simulink model "robot"  (R2021b)
settings: Solver=VariableStepAuto  StartTime=0.0  StopTime=10.0  RelTol=1e-3
settings Model: Creator=nose  LastModifiedBy=nose

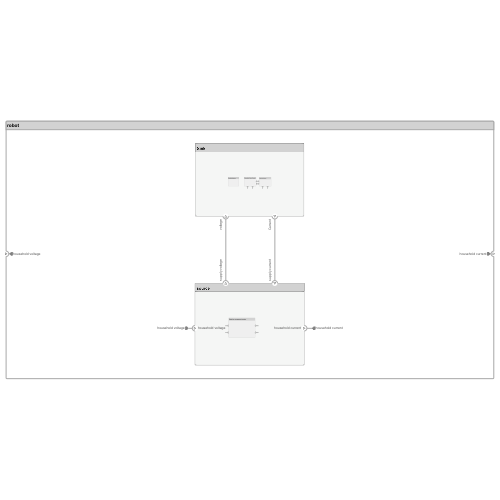
[thumbnail: Simulink's stored preview of the top-level diagram]
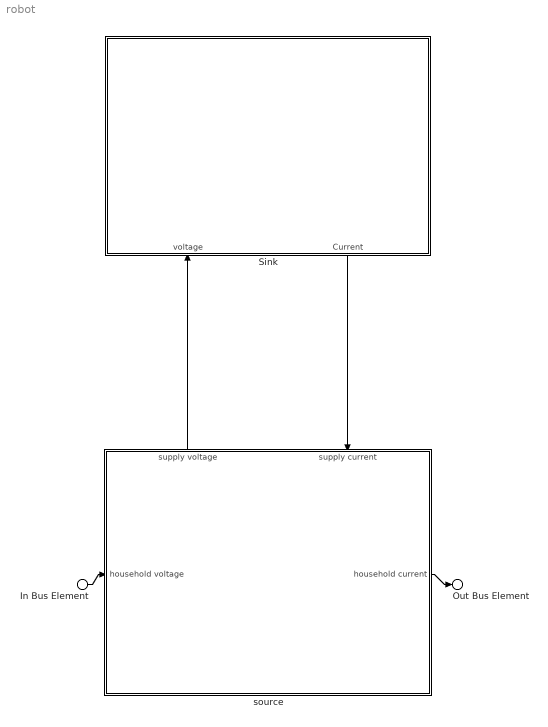
== system robot ==
  In Bus Element : Inport  PortName=household voltage
  Sink : Subsystem
      settings: PortSchema="{\"entries\":[{\"content\":{\"headerSize\":26,\"margin\":15,\"minimumSpacing\":25,\"sides\":[{\"content\":{\"connectorIds\":[]},\"type\":\"ConnectorPlacement.EquallySpacedRectSide\",\"uuid\":\"cce8d1cc-6771-426c-a0de-23a5c058ae44\"},{\"content\":{\"connectorIds\":[],\"side\":\"RIGHT\"},\"type\":\"ConnectorPlacement.EquallySpacedRectSide\",\"uuid\":\"57c46e29-2934-445f-8a04-6ff3f7f4d8fe\"},{\"content\":{\"connectorIds\":[],\"side\":\"TOP\"},\"type\":\"ConnectorPlacement.EquallySpacedRectSide\",\"uuid\":\"eb7067c1-d55e-4ae9-8630-454649e8da1e\"},{\"content\":{\"connectorIds\":[\"In1\",\"Out1\"],\"side\":\"BOTTOM\"},\"type\":\"ConnectorPlacement.EquallySpacedRectSide\",\"uuid\":\"bc61e0b0-20e7-4f9c-89f5-67eb8e0015e0\"}]},\"type\":\"ConnectorPlacement.EquallySpacedConnector\",\"uuid\":\"1a3d1b89-b469-44fc-bf92-2227b5eeb5a6\"}],\"packageUris\":[\"http://schema.mathworks.com/mf0/Connector/R2020b\"],\"version\":\"1.0\"}"
  source : Subsystem
      settings: PortSchema="{\"entries\":[{\"content\":{\"headerSize\":26,\"margin\":15,\"minimumSpacing\":25,\"sides\":[{\"content\":{\"connectorIds\":[\"In2\"]},\"type\":\"ConnectorPlacement.EquallySpacedRectSide\",\"uuid\":\"ab86f7c5-15df-4aa4-a70b-4ed2f79f5c32\"},{\"content\":{\"connectorIds\":[\"Out2\"],\"side\":\"RIGHT\"},\"type\":\"ConnectorPlacement.EquallySpacedRectSide\",\"uuid\":\"f1963fa8-65f4-4463-a82d-b8789b675b03\"},{\"content\":{\"connectorIds\":[\"Out1\",\"In1\"],\"side\":\"TOP\"},\"type\":\"ConnectorPlacement.EquallySpacedRectSide\",\"uuid\":\"01db5666-12b9-44bb-bd5a-5c24c4f58114\"}]},\"type\":\"ConnectorPlacement.EquallySpacedConnector\",\"uuid\":\"46f17ec4-de72-4b29-af46-4a561b3ef7e3\"}],\"packageUris\":[\"http://schema.mathworks.com/mf0/Connector/R2020b\"],\"version\":\"1.0\"}"
  Out Bus Element : Outport  PortName=household current
  wires:
  source/1(supply voltage) -> Sink/1(voltage)
  Sink/1(Current) -> source/1(supply current)
  In Bus Element/1 -> source/2(household voltage)
  source/2(household current) -> Out Bus Element/1

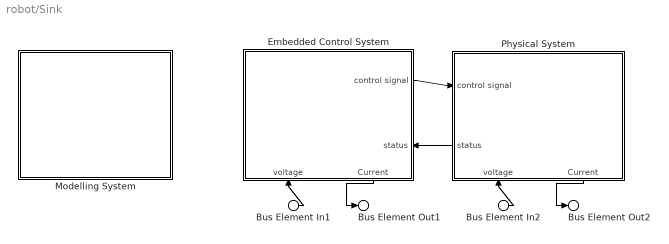
== system robot/Sink ==
  Bus Element In1 : Inport  PortName=voltage  Element=control
  Bus Element In2 : Inport  PortName=voltage  Element=physical
  Embedded Control System : Subsystem
      settings: PortSchema="{\"entries\":[{\"content\":{\"headerSize\":26,\"margin\":15,\"minimumSpacing\":25,\"sides\":[{\"content\":{\"connectorIds\":[]},\"type\":\"ConnectorPlacement.EquallySpacedRectSide\",\"uuid\":\"cce8d1cc-6771-426c-a0de-23a5c058ae44\"},{\"content\":{\"connectorIds\":[\"Out1\",\"In1\"],\"side\":\"RIGHT\"},\"type\":\"ConnectorPlacement.EquallySpacedRectSide\",\"uuid\":\"57c46e29-2934-445f-8a04-6ff3f7f4d8fe\"},{\"content\":{\"connectorIds\":[],\"side\":\"TOP\"},\"type\":\"ConnectorPlacement.EquallySpacedRectSide\",\"uuid\":\"eb7067c1-d55e-4ae9-8630-454649e8da1e\"},{\"content\":{\"connectorIds\":[\"In2\",\"Out2\"],\"side\":\"BOTTOM\"},\"type\":\"ConnectorPlacement.EquallySpacedRectSide\",\"uuid\":\"13b887ef-efdd-4ebb-88f0-3b7172777dfc\"}]},\"type\":\"ConnectorPlacement.EquallySpacedConnector\",\"uuid\":\"1a3d1b89-b469-44fc-bf92-2227b5eeb5a6\"}],\"packageUris\":[\"http://schema.mathworks.com/mf0/Connector/R2020b\"],\"version\":\"1.0\"}"
  Modelling System : Subsystem
      settings: PortSchema="{\"entries\":[{\"content\":{\"headerSize\":26,\"margin\":15,\"minimumSpacing\":25,\"sides\":[{\"content\":{\"connectorIds\":[]},\"type\":\"ConnectorPlacement.EquallySpacedRectSide\",\"uuid\":\"cce8d1cc-6771-426c-a0de-23a5c058ae44\"},{\"content\":{\"connectorIds\":[],\"side\":\"RIGHT\"},\"type\":\"ConnectorPlacement.EquallySpacedRectSide\",\"uuid\":\"57c46e29-2934-445f-8a04-6ff3f7f4d8fe\"},{\"content\":{\"connectorIds\":[],\"side\":\"TOP\"},\"type\":\"ConnectorPlacement.EquallySpacedRectSide\",\"uuid\":\"eb7067c1-d55e-4ae9-8630-454649e8da1e\"}]},\"type\":\"ConnectorPlacement.EquallySpacedConnector\",\"uuid\":\"1a3d1b89-b469-44fc-bf92-2227b5eeb5a6\"}],\"packageUris\":[\"http://schema.mathworks.com/mf0/Connector/R2020b\"],\"version\":\"1.0\"}"
  Physical System : Subsystem
      settings: PortSchema="{\"entries\":[{\"content\":{\"headerSize\":26,\"margin\":15,\"minimumSpacing\":25,\"sides\":[{\"content\":{\"connectorIds\":[\"In1\",\"Out1\"]},\"type\":\"ConnectorPlacement.EquallySpacedRectSide\",\"uuid\":\"cce8d1cc-6771-426c-a0de-23a5c058ae44\"},{\"content\":{\"connectorIds\":[],\"side\":\"RIGHT\"},\"type\":\"ConnectorPlacement.EquallySpacedRectSide\",\"uuid\":\"57c46e29-2934-445f-8a04-6ff3f7f4d8fe\"},{\"content\":{\"connectorIds\":[],\"side\":\"TOP\"},\"type\":\"ConnectorPlacement.EquallySpacedRectSide\",\"uuid\":\"eb7067c1-d55e-4ae9-8630-454649e8da1e\"},{\"content\":{\"connectorIds\":[\"In2\",\"Out2\"],\"side\":\"BOTTOM\"},\"type\":\"ConnectorPlacement.EquallySpacedRectSide\",\"uuid\":\"76e84532-edcd-4bc8-b0e9-3aa90831f893\"}]},\"type\":\"ConnectorPlacement.EquallySpacedConnector\",\"uuid\":\"1a3d1b89-b469-44fc-bf92-2227b5eeb5a6\"}],\"packageUris\":[\"http://schema.mathworks.com/mf0/Connector/R2020b\"],\"version\":\"1.0\"}"
  Bus Element Out1 : Outport  PortName=Current  Element=control
  Bus Element Out2 : Outport  PortName=Current  Element=physical
  wires:
  Bus Element In1/1 -> Embedded Control System/2(voltage)
  Bus Element In2/1 -> Physical System/2(voltage)
  Embedded Control System/2(Current) -> Bus Element Out1/1
  Physical System/2(Current) -> Bus Element Out2/1
  Embedded Control System/1(control signal) -> Physical System/1(control signal)
  Physical System/1(status) -> Embedded Control System/1(status)

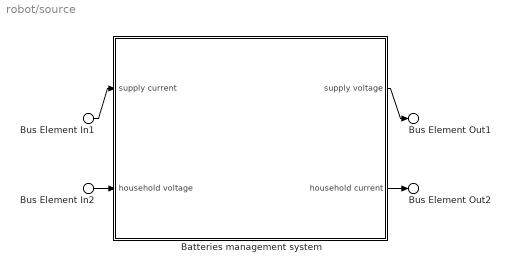
== system robot/source ==
  Bus Element In1 : Inport  PortName=supply current
  Bus Element In2 : Inport  Port=2  PortName=household voltage
  Batteries management system : Subsystem
      settings: PortSchema="{\"entries\":[{\"content\":{\"headerSize\":26,\"margin\":15,\"minimumSpacing\":25,\"sides\":[{\"content\":{\"connectorIds\":[\"In1\",\"In2\"]},\"type\":\"ConnectorPlacement.EquallySpacedRectSide\",\"uuid\":\"ab86f7c5-15df-4aa4-a70b-4ed2f79f5c32\"},{\"content\":{\"connectorIds\":[\"Out2\",\"Out1\"],\"side\":\"RIGHT\"},\"type\":\"ConnectorPlacement.EquallySpacedRectSide\",\"uuid\":\"f1963fa8-65f4-4463-a82d-b8789b675b03\"},{\"content\":{\"connectorIds\":[],\"side\":\"TOP\"},\"type\":\"ConnectorPlacement.EquallySpacedRectSide\",\"uuid\":\"01db5666-12b9-44bb-bd5a-5c24c4f58114\"},{\"content\":{\"connectorIds\":[],\"side\":\"BOTTOM\"},\"type\":\"ConnectorPlacement.EquallySpacedRectSide\",\"uuid\":\"ad04bc5b-bf31-4298-9687-69f53933a826\"}]},\"type\":\"ConnectorPlacement.EquallySpacedConnector\",\"uuid\":\"46f17ec4-de72-4b29-af46-4a561b3ef7e3\"}],\"packageUris\":[\"http://schema.mathworks.com/mf0/Connector/R2020b\"],\"version\":\"1.0\"}"
  Bus Element Out1 : Outport  PortName=supply voltage
  Bus Element Out2 : Outport  Port=2  PortName=household current
  wires:
  Bus Element In1/1 -> Batteries management system/1(supply current)
  Batteries management system/2(supply voltage) -> Bus Element Out1/1
  Bus Element In2/1 -> Batteries management system/2(household voltage)
  Batteries management system/1(household current) -> Bus Element Out2/1

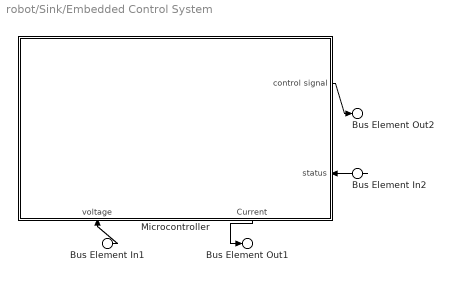
== system robot/Sink/Embedded Control System ==
  Bus Element In2 : Inport  PortName=status
  Bus Element In1 : Inport  Port=2  PortName=voltage
  Microcontroller : Subsystem
      settings: PortSchema="{\"entries\":[{\"content\":{\"headerSize\":26,\"margin\":15,\"minimumSpacing\":25,\"sides\":[{\"content\":{\"connectorIds\":[]},\"type\":\"ConnectorPlacement.EquallySpacedRectSide\",\"uuid\":\"bdb45843-8dc8-4990-9bf3-624b48549b20\"},{\"content\":{\"connectorIds\":[\"Out2\",\"In2\"],\"side\":\"RIGHT\"},\"type\":\"ConnectorPlacement.EquallySpacedRectSide\",\"uuid\":\"0a73e1fb-4df2-4d5d-a61e-038e5c52e735\"},{\"content\":{\"connectorIds\":[],\"side\":\"TOP\"},\"type\":\"ConnectorPlacement.EquallySpacedRectSide\",\"uuid\":\"48b402de-12bd-4d2a-b9ce-c931ca0ce21c\"},{\"content\":{\"connectorIds\":[\"In1\",\"Out1\"],\"side\":\"BOTTOM\"},\"type\":\"ConnectorPlacement.EquallySpacedRectSide\",\"uuid\":\"c7ff1f7c-598d-4839-a261-d2e7959d2121\"}]},\"type\":\"ConnectorPlacement.EquallySpacedConnector\",\"uuid\":\"51fa05e7-43b8-43a9-952b-69997c969bcd\"}],\"packageUris\":[\"http://schema.mathworks.com/mf0/Connector/R2020b\"],\"version\":\"1.0\"}"
  Bus Element Out2 : Outport  PortName=control signal
  Bus Element Out1 : Outport  Port=2  PortName=Current
  wires:
  Bus Element In2/1 -> Microcontroller/2(status)
  Microcontroller/2(control signal) -> Bus Element Out2/1
  Bus Element In1/1 -> Microcontroller/1(voltage)
  Microcontroller/1(Current) -> Bus Element Out1/1

== system robot/Sink/Modelling System ==

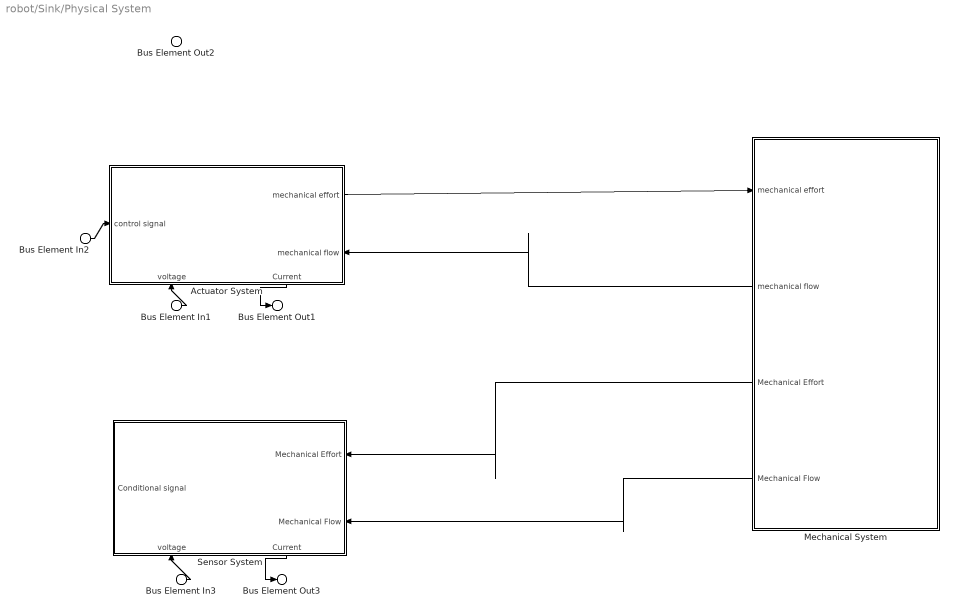
== system robot/Sink/Physical System ==
  Bus Element In2 : Inport  PortName=control signal
  Bus Element In1 : Inport  Port=2  PortName=voltage  Element=actuator
  Bus Element In3 : Inport  Port=2  PortName=voltage  Element=sensor
  Actuator System : Subsystem
      settings: PortSchema="{\"entries\":[{\"content\":{\"headerSize\":26,\"margin\":15,\"minimumSpacing\":25,\"sides\":[{\"content\":{\"connectorIds\":[\"In2\"]},\"type\":\"ConnectorPlacement.EquallySpacedRectSide\",\"uuid\":\"cce8d1cc-6771-426c-a0de-23a5c058ae44\"},{\"content\":{\"connectorIds\":[\"Out2\",\"In3\"],\"side\":\"RIGHT\"},\"type\":\"ConnectorPlacement.EquallySpacedRectSide\",\"uuid\":\"57c46e29-2934-445f-8a04-6ff3f7f4d8fe\"},{\"content\":{\"connectorIds\":[],\"side\":\"TOP\"},\"type\":\"ConnectorPlacement.EquallySpacedRectSide\",\"uuid\":\"eb7067c1-d55e-4ae9-8630-454649e8da1e\"},{\"content\":{\"connectorIds\":[\"In1\",\"Out1\"],\"side\":\"BOTTOM\"},\"type\":\"ConnectorPlacement.EquallySpacedRectSide\",\"uuid\":\"e184a07b-f7e7-418f-a075-a6148e69a320\"}]},\"type\":\"ConnectorPlacement.EquallySpacedConnector\",\"uuid\":\"1a3d1b89-b469-44fc-bf92-2227b5eeb5a6\"}],\"packageUris\":[\"http://schema.mathworks.com/mf0/Connector/R2020b\"],\"version\":\"1.0\"}"
  Mechanical System : Subsystem
      settings: PortSchema="{\"entries\":[{\"content\":{\"headerSize\":26,\"margin\":15,\"minimumSpacing\":25,\"sides\":[{\"content\":{\"connectorIds\":[\"In1\",\"Out1\",\"Out2\",\"Out3\"]},\"type\":\"ConnectorPlacement.EquallySpacedRectSide\",\"uuid\":\"cce8d1cc-6771-426c-a0de-23a5c058ae44\"},{\"content\":{\"connectorIds\":[],\"side\":\"RIGHT\"},\"type\":\"ConnectorPlacement.EquallySpacedRectSide\",\"uuid\":\"57c46e29-2934-445f-8a04-6ff3f7f4d8fe\"},{\"content\":{\"connectorIds\":[],\"side\":\"TOP\"},\"type\":\"ConnectorPlacement.EquallySpacedRectSide\",\"uuid\":\"eb7067c1-d55e-4ae9-8630-454649e8da1e\"},{\"content\":{\"connectorIds\":[],\"side\":\"BOTTOM\"},\"type\":\"ConnectorPlacement.EquallySpacedRectSide\",\"uuid\":\"4708bf5e-c359-4b7b-a4d3-6301d6aaf289\"}]},\"type\":\"ConnectorPlacement.EquallySpacedConnector\",\"uuid\":\"1a3d1b89-b469-44fc-bf92-2227b5eeb5a6\"}],\"packageUris\":[\"http://schema.mathworks.com/mf0/Connector/R2020b\"],\"version\":\"1.0\"}"
  Sensor System : Subsystem
      settings: PortSchema="{\"entries\":[{\"content\":{\"headerSize\":26,\"margin\":15,\"minimumSpacing\":25,\"sides\":[{\"content\":{\"connectorIds\":[\"Out1\"]},\"type\":\"ConnectorPlacement.EquallySpacedRectSide\",\"uuid\":\"cce8d1cc-6771-426c-a0de-23a5c058ae44\"},{\"content\":{\"connectorIds\":[\"In1\",\"In2\"],\"side\":\"RIGHT\"},\"type\":\"ConnectorPlacement.EquallySpacedRectSide\",\"uuid\":\"57c46e29-2934-445f-8a04-6ff3f7f4d8fe\"},{\"content\":{\"connectorIds\":[],\"side\":\"TOP\"},\"type\":\"ConnectorPlacement.EquallySpacedRectSide\",\"uuid\":\"eb7067c1-d55e-4ae9-8630-454649e8da1e\"},{\"content\":{\"connectorIds\":[\"In3\",\"Out2\"],\"side\":\"BOTTOM\"},\"type\":\"ConnectorPlacement.EquallySpacedRectSide\",\"uuid\":\"956056ff-9723-44b8-9837-a0ccb26e421f\"}]},\"type\":\"ConnectorPlacement.EquallySpacedConnector\",\"uuid\":\"1a3d1b89-b469-44fc-bf92-2227b5eeb5a6\"}],\"packageUris\":[\"http://schema.mathworks.com/mf0/Connector/R2020b\"],\"version\":\"1.0\"}"
  Bus Element Out2 : Outport  PortName=status
  Bus Element Out1 : Outport  Port=2  PortName=Current  Element=actuator
  Bus Element Out3 : Outport  Port=2  PortName=Current  Element=sensor
  wires:
  Bus Element In2/1 -> Actuator System/2(control signal)
  Bus Element In1/1 -> Actuator System/1(voltage)
  Actuator System/1(Current) -> Bus Element Out1/1
  Bus Element In3/1 -> Sensor System/3(voltage)
  Sensor System/2(Current) -> Bus Element Out3/1
  Actuator System/2(mechanical effort) -> Mechanical System/1(mechanical effort)
  Mechanical System/1(mechanical flow) -> Actuator System/3(mechanical flow)
  Mechanical System/3(Mechanical Flow) -> Sensor System/2(Mechanical Flow)
  Mechanical System/2(Mechanical Effort) -> Sensor System/1(Mechanical Effort)

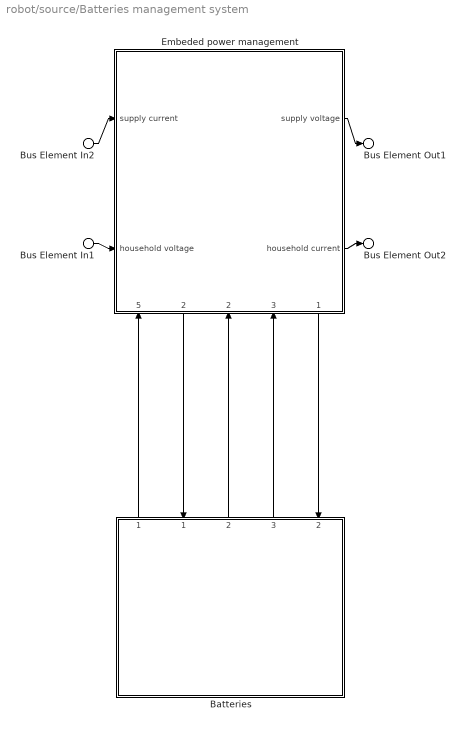
== system robot/source/Batteries management system ==
  Bus Element In2 : Inport  PortName=supply current
  Bus Element In1 : Inport  Port=2  PortName=household voltage
  Batteries : Subsystem
      settings: PortSchema="{\"entries\":[{\"content\":{\"headerSize\":26,\"margin\":15,\"minimumSpacing\":25,\"sides\":[{\"content\":{\"connectorIds\":[]},\"type\":\"ConnectorPlacement.EquallySpacedRectSide\",\"uuid\":\"ab86f7c5-15df-4aa4-a70b-4ed2f79f5c32\"},{\"content\":{\"connectorIds\":[],\"side\":\"RIGHT\"},\"type\":\"ConnectorPlacement.EquallySpacedRectSide\",\"uuid\":\"f1963fa8-65f4-4463-a82d-b8789b675b03\"},{\"content\":{\"connectorIds\":[\"Out1\",\"In1\",\"Out2\",\"Out3\",\"In2\"],\"side\":\"TOP\"},\"type\":\"ConnectorPlacement.EquallySpacedRectSide\",\"uuid\":\"01db5666-12b9-44bb-bd5a-5c24c4f58114\"},{\"content\":{\"connectorIds\":[],\"side\":\"BOTTOM\"},\"type\":\"ConnectorPlacement.EquallySpacedRectSide\",\"uuid\":\"385b722a-c9c2-490c-8613-c9d479ecdf26\"}]},\"type\":\"ConnectorPlacement.EquallySpacedConnector\",\"uuid\":\"46f17ec4-de72-4b29-af46-4a561b3ef7e3\"}],\"packageUris\":[\"http://schema.mathworks.com/mf0/Connector/R2020b\"],\"version\":\"1.0\"}"
  Embeded power management : Subsystem
      settings: PortSchema="{\"entries\":[{\"content\":{\"headerSize\":26,\"margin\":15,\"minimumSpacing\":25,\"sides\":[{\"content\":{\"connectorIds\":[\"In1\",\"In4\"]},\"type\":\"ConnectorPlacement.EquallySpacedRectSide\",\"uuid\":\"ab86f7c5-15df-4aa4-a70b-4ed2f79f5c32\"},{\"content\":{\"connectorIds\":[\"Out3\",\"Out4\"],\"side\":\"RIGHT\"},\"type\":\"ConnectorPlacement.EquallySpacedRectSide\",\"uuid\":\"f1963fa8-65f4-4463-a82d-b8789b675b03\"},{\"content\":{\"connectorIds\":[],\"side\":\"TOP\"},\"type\":\"ConnectorPlacement.EquallySpacedRectSide\",\"uuid\":\"01db5666-12b9-44bb-bd5a-5c24c4f58114\"},{\"content\":{\"connectorIds\":[\"In5\",\"Out2\",\"In2\",\"In3\",\"Out1\"],\"side\":\"BOTTOM\"},\"type\":\"ConnectorPlacement.EquallySpacedRectSide\",\"uuid\":\"1d087876-a591-45f8-ba44-eb30e0d76679\"}]},\"type\":\"ConnectorPlacement.EquallySpacedConnector\",\"uuid\":\"46f17ec4-de72-4b29-af46-4a561b3ef7e3\"}],\"packageUris\":[\"http://schema.mathworks.com/mf0/Connector/R2020b\"],\"version\":\"1.0\"}"
  Bus Element Out2 : Outport  PortName=household current
  Bus Element Out1 : Outport  Port=2  PortName=supply voltage
  wires:
  Batteries/1(control signal) -> Embeded power management/5(control signal)
  Bus Element In1/1 -> Embeded power management/4(household voltage)
  Embeded power management/4(household current) -> Bus Element Out2/1
  Embeded power management/3(supply voltage) -> Bus Element Out1/1
  Bus Element In2/1 -> Embeded power management/1(supply current)
  Embeded power management/2(charge volage) -> Batteries/1(charge volage)
  Batteries/3(discharge voltage) -> Embeded power management/3(discharge voltage)
  Embeded power management/1(discharge current) -> Batteries/2(discharge current)
  Batteries/2(charge current) -> Embeded power management/2(charge current)

== system robot/Sink/Embedded Control System/Microcontroller ==
  Bus Element In2 : Inport  PortName=voltage
  Bus Element In1 : Inport  Port=2  PortName=status
  Bus Element Out2 : Outport  PortName=Current
  Bus Element Out1 : Outport  Port=2  PortName=control signal

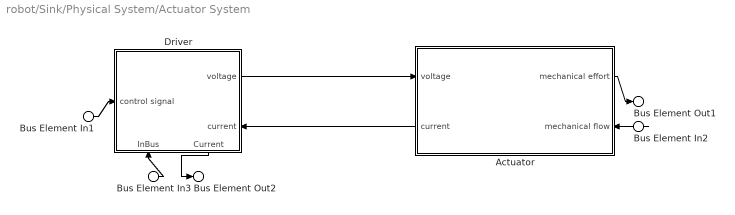
== system robot/Sink/Physical System/Actuator System ==
  Bus Element In3 : Inport  PortName=voltage
  Bus Element In1 : Inport  Port=2  PortName=control signal
  Bus Element In2 : Inport  Port=3  PortName=mechanical flow
  Actuator : Subsystem
      settings: PortSchema="{\"entries\":[{\"content\":{\"headerSize\":26,\"margin\":15,\"minimumSpacing\":25,\"sides\":[{\"content\":{\"connectorIds\":[\"In2\",\"Out2\"]},\"type\":\"ConnectorPlacement.EquallySpacedRectSide\",\"uuid\":\"cce8d1cc-6771-426c-a0de-23a5c058ae44\"},{\"content\":{\"connectorIds\":[\"Out1\",\"In1\"],\"side\":\"RIGHT\"},\"type\":\"ConnectorPlacement.EquallySpacedRectSide\",\"uuid\":\"57c46e29-2934-445f-8a04-6ff3f7f4d8fe\"},{\"content\":{\"connectorIds\":[],\"side\":\"TOP\"},\"type\":\"ConnectorPlacement.EquallySpacedRectSide\",\"uuid\":\"eb7067c1-d55e-4ae9-8630-454649e8da1e\"}]},\"type\":\"ConnectorPlacement.EquallySpacedConnector\",\"uuid\":\"1a3d1b89-b469-44fc-bf92-2227b5eeb5a6\"}],\"packageUris\":[\"http://schema.mathworks.com/mf0/Connector/R2020b\"],\"version\":\"1.0\"}"
  Driver : Subsystem
      settings: PortSchema="{\"entries\":[{\"content\":{\"headerSize\":26,\"margin\":15,\"minimumSpacing\":25,\"sides\":[{\"content\":{\"connectorIds\":[\"In3\"]},\"type\":\"ConnectorPlacement.EquallySpacedRectSide\",\"uuid\":\"cce8d1cc-6771-426c-a0de-23a5c058ae44\"},{\"content\":{\"connectorIds\":[\"Out2\",\"In2\"],\"side\":\"RIGHT\"},\"type\":\"ConnectorPlacement.EquallySpacedRectSide\",\"uuid\":\"57c46e29-2934-445f-8a04-6ff3f7f4d8fe\"},{\"content\":{\"connectorIds\":[],\"side\":\"TOP\"},\"type\":\"ConnectorPlacement.EquallySpacedRectSide\",\"uuid\":\"eb7067c1-d55e-4ae9-8630-454649e8da1e\"},{\"content\":{\"connectorIds\":[\"In1\",\"Out1\"],\"side\":\"BOTTOM\"},\"type\":\"ConnectorPlacement.EquallySpacedRectSide\",\"uuid\":\"0c06931e-5f4b-49d1-94e0-070c126ce7a1\"}]},\"type\":\"ConnectorPlacement.EquallySpacedConnector\",\"uuid\":\"1a3d1b89-b469-44fc-bf92-2227b5eeb5a6\"}],\"packageUris\":[\"http://schema.mathworks.com/mf0/Connector/R2020b\"],\"version\":\"1.0\"}"
  Bus Element Out2 : Outport  PortName=Current
  Bus Element Out1 : Outport  Port=2  PortName=mechanical effort
  wires:
  Bus Element In1/1 -> Driver/3(control signal)
  Driver/2(voltage) -> Actuator/2(voltage)
  Actuator/2(current) -> Driver/2(current)
  Actuator/1(mechanical effort) -> Bus Element Out1/1
  Bus Element In2/1 -> Actuator/1(mechanical flow)
  Driver/1(Current) -> Bus Element Out2/1
  Bus Element In3/1 -> Driver/1(InBus)

== system robot/Sink/Physical System/Mechanical System ==
  Bus Element In1 : Inport  PortName=mechanical effort
  Bus Element Out1 : Outport  PortName=mechanical flow
  Bus Element Out3 : Outport  Port=2  PortName=Mechanical Effort
  Bus Element Out2 : Outport  Port=3  PortName=Mechanical Flow

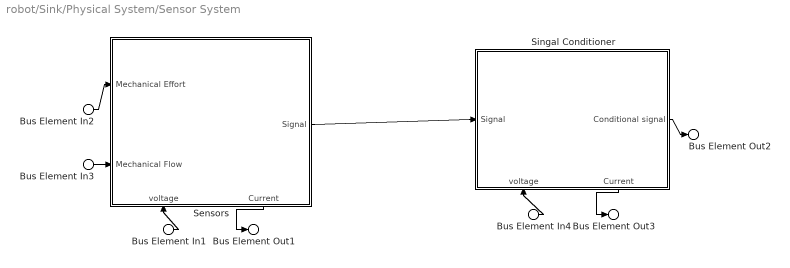
== system robot/Sink/Physical System/Sensor System ==
  Bus Element In2 : Inport  PortName=Mechanical Effort
  Bus Element In3 : Inport  Port=2  PortName=Mechanical Flow
  Bus Element In1 : Inport  Port=3  PortName=voltage
  Bus Element In4 : Inport  Port=3  PortName=voltage
  Sensors : Subsystem
      settings: PortSchema="{\"entries\":[{\"content\":{\"headerSize\":26,\"margin\":15,\"minimumSpacing\":25,\"sides\":[{\"content\":{\"connectorIds\":[\"In2\",\"In3\"]},\"type\":\"ConnectorPlacement.EquallySpacedRectSide\",\"uuid\":\"cce8d1cc-6771-426c-a0de-23a5c058ae44\"},{\"content\":{\"connectorIds\":[\"Out1\"],\"side\":\"RIGHT\"},\"type\":\"ConnectorPlacement.EquallySpacedRectSide\",\"uuid\":\"57c46e29-2934-445f-8a04-6ff3f7f4d8fe\"},{\"content\":{\"connectorIds\":[],\"side\":\"TOP\"},\"type\":\"ConnectorPlacement.EquallySpacedRectSide\",\"uuid\":\"eb7067c1-d55e-4ae9-8630-454649e8da1e\"},{\"content\":{\"connectorIds\":[\"In1\",\"Out2\"],\"side\":\"BOTTOM\"},\"type\":\"ConnectorPlacement.EquallySpacedRectSide\",\"uuid\":\"a18217dc-0b35-4565-b7f0-461a45ac447c\"}]},\"type\":\"ConnectorPlacement.EquallySpacedConnector\",\"uuid\":\"1a3d1b89-b469-44fc-bf92-2227b5eeb5a6\"}],\"packageUris\":[\"http://schema.mathworks.com/mf0/Connector/R2020b\"],\"version\":\"1.0\"}"
  Singal Conditioner : Subsystem
      settings: PortSchema="{\"entries\":[{\"content\":{\"headerSize\":26,\"margin\":15,\"minimumSpacing\":25,\"sides\":[{\"content\":{\"connectorIds\":[\"In2\"]},\"type\":\"ConnectorPlacement.EquallySpacedRectSide\",\"uuid\":\"cce8d1cc-6771-426c-a0de-23a5c058ae44\"},{\"content\":{\"connectorIds\":[\"Out2\"],\"side\":\"RIGHT\"},\"type\":\"ConnectorPlacement.EquallySpacedRectSide\",\"uuid\":\"57c46e29-2934-445f-8a04-6ff3f7f4d8fe\"},{\"content\":{\"connectorIds\":[],\"side\":\"TOP\"},\"type\":\"ConnectorPlacement.EquallySpacedRectSide\",\"uuid\":\"eb7067c1-d55e-4ae9-8630-454649e8da1e\"},{\"content\":{\"connectorIds\":[\"In1\",\"Out1\"],\"side\":\"BOTTOM\"},\"type\":\"ConnectorPlacement.EquallySpacedRectSide\",\"uuid\":\"e0b4d8d5-91a9-4ade-ae6c-6b33a0b902f9\"}]},\"type\":\"ConnectorPlacement.EquallySpacedConnector\",\"uuid\":\"1a3d1b89-b469-44fc-bf92-2227b5eeb5a6\"}],\"packageUris\":[\"http://schema.mathworks.com/mf0/Connector/R2020b\"],\"version\":\"1.0\"}"
  Bus Element Out2 : Outport  PortName=Conditional signal
  Bus Element Out1 : Outport  Port=2  PortName=Current  Element=sensor
  Bus Element Out3 : Outport  Port=2  PortName=Current  Element=signal condioner
  wires:
  Bus Element In2/1 -> Sensors/2(Mechanical Effort)
  Bus Element In3/1 -> Sensors/3(Mechanical Flow)
  Bus Element In1/1 -> Sensors/1(voltage)
  Singal Conditioner/2(Conditional signal) -> Bus Element Out2/1
  Sensors/1(Signal) -> Singal Conditioner/2(Signal)
  Bus Element In4/1 -> Singal Conditioner/1(voltage)
  Sensors/2(Current) -> Bus Element Out1/1
  Singal Conditioner/1(Current) -> Bus Element Out3/1

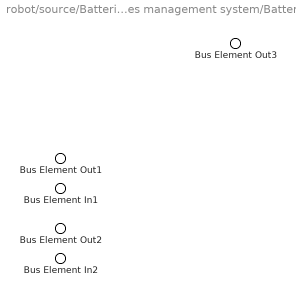
== system robot/source/Batteries management system/Batteries ==
  Bus Element In1 : Inport  PortName=charge volage
  Bus Element In2 : Inport  Port=2  PortName=discharge current
  Bus Element Out1 : Outport  PortName=control signal
  Bus Element Out3 : Outport  Port=2  PortName=charge current
  Bus Element Out2 : Outport  Port=3  PortName=discharge voltage

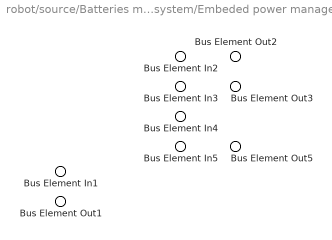
== system robot/source/Batteries management system/Embeded power management ==
  Bus Element In3 : Inport  PortName=supply current
  Bus Element In5 : Inport  Port=2  PortName=charge current
  Bus Element In4 : Inport  Port=3  PortName=discharge voltage
  Bus Element In2 : Inport  Port=4  PortName=household voltage
  Bus Element In1 : Inport  Port=5  PortName=control signal
  Bus Element Out5 : Outport  PortName=discharge current
  Bus Element Out3 : Outport  Port=2  PortName=charge volage
  Bus Element Out2 : Outport  Port=3  PortName=supply voltage
  Bus Element Out1 : Outport  Port=4  PortName=household current

== system robot/Sink/Physical System/Actuator System/Actuator ==
  Bus Element In2 : Inport  PortName=mechanical flow
  Bus Element In1 : Inport  Port=2  PortName=voltage
  Bus Element Out2 : Outport  PortName=mechanical effort
  Bus Element Out1 : Outport  Port=2  PortName=current

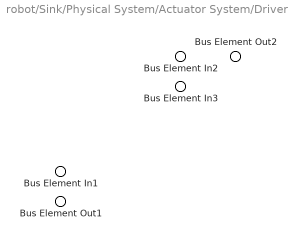
== system robot/Sink/Physical System/Actuator System/Driver ==
  Bus Element In3 : Inport  PortName=InBus
  Bus Element In2 : Inport  Port=2  PortName=current
  Bus Element In1 : Inport  Port=3  PortName=control signal
  Bus Element Out2 : Outport  PortName=Current
  Bus Element Out1 : Outport  Port=2  PortName=voltage

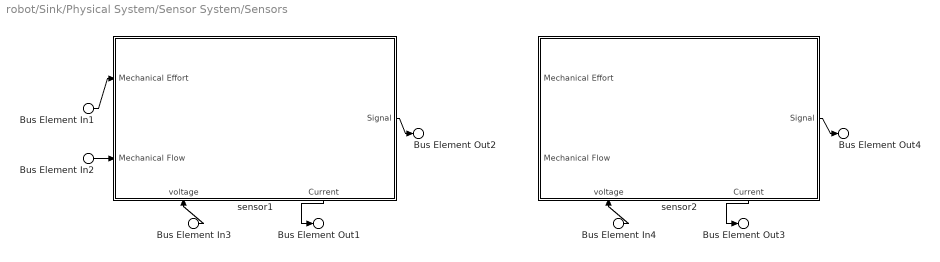
== system robot/Sink/Physical System/Sensor System/Sensors ==
  Bus Element In3 : Inport  PortName=voltage
  Bus Element In4 : Inport  PortName=voltage
  Bus Element In1 : Inport  Port=2  PortName=Mechanical Effort
  Bus Element In2 : Inport  Port=3  PortName=Mechanical Flow
  sensor1 : Subsystem
      settings: PortSchema="{\"entries\":[{\"content\":{\"headerSize\":26,\"margin\":15,\"minimumSpacing\":25,\"sides\":[{\"content\":{\"connectorIds\":[\"In2\",\"In3\"]},\"type\":\"ConnectorPlacement.EquallySpacedRectSide\",\"uuid\":\"bdb45843-8dc8-4990-9bf3-624b48549b20\"},{\"content\":{\"connectorIds\":[\"Out1\"],\"side\":\"RIGHT\"},\"type\":\"ConnectorPlacement.EquallySpacedRectSide\",\"uuid\":\"0a73e1fb-4df2-4d5d-a61e-038e5c52e735\"},{\"content\":{\"connectorIds\":[],\"side\":\"TOP\"},\"type\":\"ConnectorPlacement.EquallySpacedRectSide\",\"uuid\":\"48b402de-12bd-4d2a-b9ce-c931ca0ce21c\"},{\"content\":{\"connectorIds\":[\"In1\",\"Out2\"],\"side\":\"BOTTOM\"},\"type\":\"ConnectorPlacement.EquallySpacedRectSide\",\"uuid\":\"464871b1-3f5f-4d78-8f6a-613e90867034\"}]},\"type\":\"ConnectorPlacement.EquallySpacedConnector\",\"uuid\":\"51fa05e7-43b8-43a9-952b-69997c969bcd\"}],\"packageUris\":[\"http://schema.mathworks.com/mf0/Connector/R2020b\"],\"version\":\"1.0\"}"
  sensor2 : Subsystem
      settings: PortSchema="{\"entries\":[{\"content\":{\"headerSize\":26,\"margin\":15,\"minimumSpacing\":25,\"sides\":[{\"content\":{\"connectorIds\":[\"In2\",\"In3\"]},\"type\":\"ConnectorPlacement.EquallySpacedRectSide\",\"uuid\":\"bdb45843-8dc8-4990-9bf3-624b48549b20\"},{\"content\":{\"connectorIds\":[\"Out1\"],\"side\":\"RIGHT\"},\"type\":\"ConnectorPlacement.EquallySpacedRectSide\",\"uuid\":\"0a73e1fb-4df2-4d5d-a61e-038e5c52e735\"},{\"content\":{\"connectorIds\":[],\"side\":\"TOP\"},\"type\":\"ConnectorPlacement.EquallySpacedRectSide\",\"uuid\":\"48b402de-12bd-4d2a-b9ce-c931ca0ce21c\"},{\"content\":{\"connectorIds\":[\"In1\",\"Out2\"],\"side\":\"BOTTOM\"},\"type\":\"ConnectorPlacement.EquallySpacedRectSide\",\"uuid\":\"464871b1-3f5f-4d78-8f6a-613e90867034\"}]},\"type\":\"ConnectorPlacement.EquallySpacedConnector\",\"uuid\":\"51fa05e7-43b8-43a9-952b-69997c969bcd\"}],\"packageUris\":[\"http://schema.mathworks.com/mf0/Connector/R2020b\"],\"version\":\"1.0\"}"
  Bus Element Out2 : Outport  PortName=Signal  Element=sensor1
  Bus Element Out4 : Outport  PortName=Signal  Element=sensor2
  Bus Element Out1 : Outport  Port=2  PortName=Current  Element=sensor1
  Bus Element Out3 : Outport  Port=2  PortName=Current  Element=sensor2
  wires:
  Bus Element In1/1 -> sensor1/2(Mechanical Effort)
  Bus Element In2/1 -> sensor1/3(Mechanical Flow)
  Bus Element In3/1 -> sensor1/1(voltage)
  sensor1/1(Signal) -> Bus Element Out2/1
  Bus Element In4/1 -> sensor2/1(voltage)
  sensor1/2(Current) -> Bus Element Out1/1
  sensor2/2(Current) -> Bus Element Out3/1
  sensor2/1(Signal) -> Bus Element Out4/1

== system robot/Sink/Physical System/Sensor System/Singal Conditioner ==
  Bus Element In2 : Inport  PortName=voltage
  Bus Element In1 : Inport  Port=2  PortName=Signal
  Bus Element Out3 : Outport  PortName=Current
  Bus Element Out1 : Outport  Port=2  PortName=Conditional signal

== system robot/Sink/Physical System/Sensor System/Sensors/sensor1 ==
  Bus Element In3 : Inport  PortName=voltage
  Bus Element In1 : Inport  Port=2  PortName=Mechanical Effort
  Bus Element In2 : Inport  Port=3  PortName=Mechanical Flow
  Bus Element Out2 : Outport  PortName=Signal
  Bus Element Out1 : Outport  Port=2  PortName=Current

== system robot/Sink/Physical System/Sensor System/Sensors/sensor2 ==
  Bus Element In3 : Inport  PortName=voltage
  Bus Element In1 : Inport  Port=2  PortName=Mechanical Effort
  Bus Element In2 : Inport  Port=3  PortName=Mechanical Flow
  Bus Element Out2 : Outport  PortName=Signal
  Bus Element Out1 : Outport  Port=2  PortName=Current
